simulink library "Library_ASK"  (R2018b)
settings: Solver=VariableStepAuto  StartTime=0.0  StopTime=10.0  RelTol=1e-3  EnableMultiTasking=on
undefined symbols (not defined in the file): akt_2GTR_az_HA, akt_2GTR_az_VA, akt_2GTR_rn_HA, akt_2GTR_rn_VA, akt_GTR_az_HA, akt_GTR_az_VA, akt_GTR_rn_HA, akt_GTR_rn_VA, alpha, b_zahn, beta_b, breakpointset, choose_ulg, DiscIntNeverNeededParam, eps_1, eps_2, eps_alpha, eta_aa, eta_Kegel_max, Fx_LSD_max, Fx_mUELG_max, i_DF, i_Kegelrad_OD, i_TRM_G1_HA, i_TRM_G1_VA, i_TRM_G2_HA, i_TRM_G2_VA, i_TRM_HA, i_TRM_Stufe_1_HA, i_TRM_Stufe_1_VA, i_TRM_Stufe_2_HA, i_TRM_Stufe_2_VA, i_TRM_VA, M_Cl_LSD_max, M_Cl_mUELG_max, M_EM_max, M_Kupplung_mUELG_Schlepp, mu_cl_LSD, mu_cl_mUELG, n_EM_max, n_Stufen_TRM_HA, n_Stufen_TRM_VA, ndyn_oil, nreib_LSD, nreib_mUELG, par_MDT, par_VEH, Ra, rm_LSD, rm_mUELG, select_Traktion_split, stepsize, wkg_Diff_mUELG, wkg_GTR, X_L, z_atts, z_ayc, z_ayc_lr, z_ayc_rl
libraries: simulink x23, $bdroot x6
(part 4 of 4)

== matlab function Library_ASK/Elektrisches Überlagerungsgetriebe VA/MATLAB Function ==
  data: eta_Steuer input; M_RW input; M_LW input; M_Rad_rechts output; M_ein input; M_Rad_links output; P_Verlust_ges output; P_Steuer output; nri input; nli input; M_Steuer output; n_Steuer output; eta_eUELG output; M_Steuer_max input; i12_I input; i12_II input; i12_III input; i12_IV input; iVTV_1 input; iVTV_2 input; eta12_I input; eta12_II input; eta12_III input; eta12_IV input; etaVTV_1 input; etaVTV_2 input
 function [M_Rad_rechts, M_Rad_links, P_Verlust_ges, P_Steuer, M_Steuer, n_Steuer, eta_eUELG] = eUELG(eta_Steuer, M_RW, M_LW, M_ein, nri, nli, M_Steuer_max, i12_I, i12_II, i12_III, i12_IV, iVTV_1, iVTV_2, eta12_I, eta12_II, eta12_III, eta12_IV, etaVTV_1, etaVTV_2)
%% Übersicht
%verlagert das TV-Moment um, Versionsstand: 05.05.2017 nach evaleuelgeta_V3
%M_TV: verlagertes Moment
%nri: Ist-Drehzahl rechtes Rad
%nli: Ist-Drehzahl linkes Rad
%% Drehzahlen

%besonders n_Steuer mit dessen korrektem VZ
%Stufe I
n1_I = 0;
ns_I = nri;
n2_I = nri*(1-1/i12_I);

%Stufe II
n2_II = n2_I;
ns_II = (nri-nli*(1-i12_III))/i12_III;
if n2_II == 0 && ns_II == 0             %Stillstand
    n1_II = 0;
elseif n2_II == 0 && ns_II ~= 0         %Zweiwellenbetrieb von II
    n1_II = ns_II*(1-i12_II);
else                                    %Dreiwellenbetrieb von II
    n1_II = n2_II*((nri-nli*(1-i12_III))/(i12_III*nri*(1-1/i12_I))*(1-i12_II)+i12_II);
end
n_Steuer = n1_II*iVTV_1*iVTV_2;

%Stufe III
n1_III = nri;
ns_III = nli;
%n2_III = (nri-nli*(1-i12_III))/i12_III;

%Stufe IV
n1_IV = nri;
ns_IV = nli;
n2_IV = 0.5*(nli+nri);                 %gilt nur für i12_IV = 2!
%n2_IV = (nli/i12_IV)*(nri/nli-1+i12_IV)%alter Ausdruck, kann nan
%produzieren
%% Vorbereitung
%Verlagerungsrichtung und Kurve evaluieren
[ltr, ~] = eval_Verlagerungsrichtung(M_RW, M_LW, M_ein);
% M_TV_Wunsch = abs(M_LW-M_RW);
lk = eval_Kurve(nli, nri);

%Gewünschte Verlagerungsrichtung einstellen und Vorzeichen bekommen
% if M_TV_Wunsch <= 70
%     if nli > nri
%         sign_M_Steuer = 1;
%     elseif nli < nri
%         sign_M_Steuer = -1;
%     else
%         sign_M_Steuer = 0;
%     end
% else
%     if ltr == 1
%         sign_M_Steuer = -1;
%     elseif rtl == 1
%         sign_M_Steuer = 1;
%     else
%         sign_M_Steuer = 0;
%     end
% end

%Vorzeichen von M1_IV und damit w1_IV bestimmen
sign_M1_IV = sign(-M_ein/i12_IV);
w1_IV = sign(sign_M1_IV*(n1_IV - ns_IV));

%k4
k4 = i12_IV*eta12_IV^w1_IV;

%kritisches Verlagerungsmoment bestimmen (Nullstellensuche)
delta_M_krit = M_ein*(2/k4-1);

%sign_M_Steuer bestimmen
sign_M_Steuer = set_sign_M_Steuer(M_ein,M_LW,M_RW,nli,nri,delta_M_krit);

%w1_II ausrechnen
w1_II = sign(sign_M_Steuer*(n1_II - ns_II));

%Vorzeichen von M1_I und damit w1_I bestimmen
sign_M1_I = sign(-sign_M_Steuer*i12_II/i12_I);
w1_I = sign(sign_M1_I*(n1_I - ns_I));

%Vorzeichen von M1_III und damit w1_III bestimmen
sign_M1_III = sign(sign_M_Steuer*sign(1-i12_II*eta12_II^w1_II)*-sign(i12_III));
w1_III = sign(sign_M1_III*(n1_III - ns_III));

%% k1-3
k1 = i12_I*eta12_I^w1_I;
k2 = i12_II*eta12_II^w1_II;
k3 = i12_III*eta12_III^w1_III;

%% Betrag von M1_II exakt bestimmen:
%Die Unterscheidung nach M_ein fällt weg, da danach schon ltr bestimmt wird
mvh_TV_ex = (1-k2)*((2-k3)/k3)-k2*((1-k1)/k1);
% if ltr == 1
%         M1_II_ex = (M_TV_Wunsch-M_ein*(2/k4-1))/(mvh_TV_ex);
% else
%         M1_II_ex = (M_TV_Wunsch+M_ein*(2/k4-1))/(mvh_TV_ex);
% end
M1_II_ex = ((M_LW-M_RW)-M_ein*(2/k4-1))/(mvh_TV_ex);
%% Vorzeichen von M1_II bestimmen und Vorstufe berücksichtigen

%Modus berechnen
if sign(sign_M_Steuer*n_Steuer) == -1
    exp = -1;
else
    exp = 1;
end

%korrekten Wert berechnen und korrektes VZ zuweisen
M_Steuer = sign_M_Steuer*abs(M1_II_ex)/(iVTV_1*iVTV_2*(etaVTV_1*etaVTV_2)^exp);

%falls notwendig, Begrenzung des Betrags auf den maximalen
if abs(M_Steuer) > M_Steuer_max
     M_Steuer = M_Steuer_max*sign_M_Steuer;
end

%finales M1_II ausrechnen für die weitere Berechnung
M1_II = M_Steuer*iVTV_1*iVTV_2*(etaVTV_1*etaVTV_2)^exp;

%% Momente
M2_IV = M_ein;      %ACHTUNG M_ein ist nach der Vorstufe
MS_IV = M2_IV*(1/k4-1);
M1_IV = -M2_IV/k4;

%M1_II = M1_II;
%M2_II = M1_II*-k2;
%MS_II = -M2_II-M1_II;

MS_III = M1_II*(1-k2)*(1/k3-1);
M1_III = M1_II*(1-k2)*(1/k3-1)*(1/(k3-1));
%M2_III = -MS_II;

%M2_I = -M2_II;
%M1_I = -M2_I/k1;
MS_I = M1_II*k2*(1/k1-1);
%% Radmomente
M_Rad_links = MS_IV + MS_III;
M_Rad_rechts = MS_I + M1_III + M1_IV;
%% Leistung Steuermaschine (auskommentiert weil nicht benötigt)
P_Steuer = M_Steuer*n_Steuer/eta_Steuer;   %aus der Batterie entnommene Steuerleistung
%P_Verlust_eUELG_Steuer = P_Steuer - n_Steuer*M_Steuer; %entnommene minus verwendete Leistung
%% WKG Kennfeldmethode
%Es wird der reine Umlaufwirkungsgrad der Stufe IV mit dem
%Kennfeldwirkungsgrad der TV - Stufe multipliziert.
% [mot_ein, mot_1IV, mot_sIV, gen_ein, gen_1IV, gen_sIV] = eval_Betriebsmodus_IV(M2_IV, M1_IV, MS_IV, n2_IV, n1_IV, ns_IV);
% P_ein_IV = mot_ein*M_ein*n2_IV + mot_1IV*M1_IV*n1_IV + mot_sIV*MS_IV*ns_IV;
% P_aus_IV = gen_ein*M_ein*n2_IV + gen_1IV*M1_IV*n1_IV + gen_sIV*MS_IV*ns_IV;
% if P_aus_IV == 0 && P_ein_IV == 0
%     eta_IV = 1;
% elseif abs(P_ein_IV) < 0.1
%     eta_IV = 1;
% else
%     eta_IV = -P_aus_IV/P_ein_IV;
% end

% if  M_ein >= 0
%     if lk == 1
%         if ltr == 1
%             eta_Kennfeld = eta_TV_ltr_lk;
%         else
%             eta_Kennfeld = eta_TV_rtl_lk;
%         end
%     else
%         if ltr == 1
%             eta_Kennfeld = eta_TV_ltr_rk;
%         else
%             eta_Kennfeld = eta_TV_rtl_rk;
%         end
%     end
% else
%     if lk == 1
%         if ltr == 1
%             eta_Kennfeld = eta_TV_ltr_lk_G;
%         else
%             eta_Kennfeld = eta_TV_rtl_lk_G;
%         end
%     else
%         if ltr == 1
%             eta_Kennfeld = eta_TV_ltr_rk_G;
%         else
%             eta_Kennfeld = eta_TV_rtl_rk_G;
%         end
%     end
% end
% eta_eUELG = eta_IV*eta_Kennfeld;
%% WKG ohne Kennfelder
[mot_ein, mot_Steuer, mot_rechts, mot_links, gen_ein, gen_Steuer, gen_rechts, gen_links] = eval_Betriebsmodus(M2_IV, M_Steuer, M_Rad_rechts, M_Rad_links, n2_IV, n_Steuer, n1_IV, ns_IV);
P_ein = mot_ein*M2_IV*n2_IV + mot_Steuer*M_Steuer*n_Steuer + mot_rechts*M_Rad_rechts*n1_IV + mot_links*M_Rad_links*ns_IV;
P_aus = gen_ein*M2_IV*n2_IV + gen_Steuer*M_Steuer*n_Steuer + gen_rechts*M_Rad_rechts*n1_IV + gen_links*M_Rad_links*ns_IV;
if P_aus == 0 && P_ein == 0
    eta_eUELG = 1;
    P_Verlust_ges = 0;
elseif abs(P_ein) < 0.1
    eta_eUELG = 1;
    P_Verlust_ges = 0;
else
    eta_eUELG = -P_aus/P_ein;
    P_Verlust_ges = (1-eta_eUELG)*P_ein;
end


end

 %% Momentenverlagerung alte Methode
% 
% if mot == 1
%     if nli > nri
%         M_Rad_links = M_D + 0.5*M_TV;
%         M_Rad_rechts = M_D - 0.5*M_TV;
%         w1 = -1; w2 = 1; w3 = 1; w4 = -1;
%     else
%         M_Rad_links = M_D - 0.5*M_TV; %der Fall nli=nri tritt nicht auf, da mot == 1
%         M_Rad_rechts = M_D + 0.5*M_TV;
%         w1 = 1; w2 = -1; w3 = 1; w4 = 1;
%     end
% elseif gen == 1
%         if nli > nri
%             M_Rad_links = M_D + 0.5*M_TV;
%             M_Rad_rechts = M_D - 0.5*M_TV;
%             w1 = 1; w2 = -1; w3 = -1; w4 = 1;
%         else
%             M_Rad_links = M_D - 0.5*M_TV; %der Fall nli=nri tritt nicht auf, da gen == 1
%             M_Rad_rechts = M_D + 0.5*M_TV;
%             w1 = -1; w2 = +1; w3 = -1; w4 = -1;
%         end
% else
%         M_Rad_links = M_D;
%         M_Rad_rechts = M_D;
%         w1 = 0; w2 = 0; w3 = 0; w4 = 0;
% end

== matlab function Library_ASK/Limited Slip Differential/MATLAB Function ==
  data: eta_Diff_LSD input; M_ein input; sign_MTV input; M_Rad_rechts output; M_Kupplung input; n_ein input; nri input; nli input; M_Rad_links output; P_V_LSD output; eta_LSD output
function [M_Rad_rechts, M_Rad_links, P_V_LSD, eta_LSD] = LSD(eta_Diff_LSD, M_ein, sign_MTV, M_Kupplung, n_ein, nri, nli)

%weil es nur eine Kupplung gibt und die Momentenverteilungsrichtung sich
%automatisch ergibt, reicht es, einfach den Betrag des TV-Momentes (=Kupplungsmoment) zu
%nehmen und die Kupplung danach zu regeln. Das TV-Moment wird einfach da
%addiert, wo die Räder langsamer drehen.

%Versuch: Kupplung nur ab bestimmter Schwelle schließen (1,05fache
%Drehgeschwindigkeit)
%kombiversion

M_D = M_ein*eta_Diff_LSD/2;
%% Logik für übertragbares Maximalmoment
%maximal übertragbares Moment in der Kupplung: hängt von den Drehzahlen und
%der Kupplung selbst ab; M_Cl_grenz ist das Moment, was betriebsabhängig
%wirklich verlagert werden kann
% M_Cl_max = 200;
% if abs(nli-nri) < 20
%     M_Cl_grenz = ((abs(nli-nri))/20)*M_Cl_max;
% else
%     M_Cl_grenz = M_Cl_max;
% end
% 
% if M_TV > M_Cl_grenz
%     M_TV = M_Cl_grenz;
% end

%% Ausführungsbedingung: Wunschverlagerungsrichtung soll nicht konterkariert werden
% %sign_MTV = links-rechts
% if (sign_MTV > 0 && nli < nri)|| (sign_MTV < 0 && nri < nli)
%     okay = 1;
% else
%     okay = 0;
% end
%% Verlagerungslogik
if (nri > nli) % && okay == 1
    M_Rad_rechts = M_D - M_Kupplung;
    M_Rad_links = M_D + M_Kupplung;
elseif (nri < nli) % && okay == 1
      M_Rad_rechts = M_D + M_Kupplung;
      M_Rad_links = M_D - M_Kupplung;
else
    M_Rad_rechts = M_D;
    M_Rad_links = M_D;
end

%% Verluste

P_V_Cl = 2*pi*M_Kupplung*abs(nri-nli);
P_V_Verz = 2*pi*M_ein*n_ein*(1-eta_Diff_LSD);
P_V_LSD = P_V_Cl + P_V_Verz;
P_ein = M_ein*n_ein;
P_aus = M_Rad_rechts*nri + M_Rad_links*nli;
eta_LSD = P_aus/P_ein;

end

== matlab function Library_ASK/Limited Slip Differential/MATLAB Function1 ==
  data: sign_MTV input; okay output; nri input; nli input
function okay = execute_clutch(sign_MTV, nri, nli)
%entscheidet, ob die Kupplung geschlossen wird oder nicht

if (sign_MTV > 0 && nli < nri)|| (sign_MTV < 0 && nri < nli)
    okay = 1;
else
    okay = 0;
end

end

== matlab function Library_ASK/mechanisches Ueberlagerungsgetriebe/MATLAB Function1 ==
  data: M_RW input; okay_CL output; okay_CR output; M_LW input; nri input; nli input; i_DF input
function [okay_CL, okay_CR] = execute_clutch_mUELG(M_RW, M_LW, nri, nli, i_DF)
%entscheidet, ob die Kupplungen aktuiert werden

[ltr, rtl] = eval_Verlagerungsrichtung(M_RW, M_LW);

n_cl_s1 = nli;
n_cl_s2 = nri*i_DF;
n_cr_s1 = nri;
n_cr_s2 = nli*i_DF;

if (ltr == 1 && n_cr_s1 ~= n_cr_s2)         %nicht kuppeln wenn die Hälften gleich schnell drehen
    okay_CL = 0;
    okay_CR = 1;
elseif (rtl == 1 && n_cl_s1 ~= n_cl_s2)
    okay_CL = 1;
    okay_CR = 0;
else
    okay_CL = 0;
    okay_CR = 0;
end

== matlab function Library_ASK/mechanisches Ueberlagerungsgetriebe/Transmission Choice/MATLAB Function ==
  data: M_RW input; M_LW input; M_Clutch output; i_DF input; z_ayc_lr input; z_ayc_rl input; z_atts input; choose_ulg input
function M_Clutch  = config_ULG(M_RW, M_LW, i_DF, z_ayc_lr, z_ayc_rl, z_atts, choose_ulg)
%calculates clutch torque from desired vectoring torque dependent on the
%cosen kind of mech. ÜLG: Prinzipskizze (0), Mitsubishi AYC (1), Mitsubishi Super AYC (2) and Honda
%ATTS (3)

M_TV = abs(M_RW-M_LW);

[ltr, rtl] = eval_Verlagerungsrichtung(M_RW, M_LW);
if ltr == 1
    z_ayc = z_ayc_lr;
elseif rtl == 1
    z_ayc = z_ayc_rl;
else
    z_ayc = 0;
end

switch choose_ulg
    case 0
        M_Clutch = M_TV*i_DF/(i_DF+1);
    case 1
        M_Clutch = M_TV;
    case 2
        M_Clutch = M_TV/(z_ayc+1);
    case 3
        M_Clutch = M_TV/(2*(z_atts+1));  %Hier ist M_Clutch eine Bremse
    otherwise
        M_Clutch = 0;
end

== matlab function Library_ASK/mechanisches Ueberlagerungsgetriebe/MATLAB Function2 ==
  data: M_Kupplung input; M_TV output; i_DF input; z_ayc input; z_atts input; choose_ulg input
function M_TV = reverse_config(M_Kupplung, i_DF, z_ayc, z_atts, choose_ulg)
%rechnet vom tatsächlichen M_Kupplung zurück auf MTV, damit das nicht in der Hauptfunktion drinstehen
%muss

switch choose_ulg
    case 0
        M_TV = M_Kupplung(1-1/i_DF);
    case 1
        M_TV = M_Kupplung;
    case 2
        M_TV = M_Kupplung(z_ayc+1);
    case 3
        M_TV = 2*M_Kupplung*(1+z_atts);
    otherwise
        M_TV = 0;
end

end

== matlab function Library_ASK/Elektrisches Überlagerungsgetriebe HA/MATLAB Function ==
  data: eta_Steuer input; M_RW input; M_LW input; M_Rad_rechts output; M_ein input; M_Rad_links output; P_Verlust_ges output; P_Steuer output; nri input; nli input; M_Steuer output; n_Steuer output; eta_eUELG output; M_Steuer_max input; i12_I input; i12_II input; i12_III input; i12_IV input; iVTV_1 input; iVTV_2 input; eta12_I input; eta12_II input; eta12_III input; eta12_IV input; etaVTV_1 input; etaVTV_2 input
 function [M_Rad_rechts, M_Rad_links, P_Verlust_ges, P_Steuer, M_Steuer, n_Steuer, eta_eUELG] = eUELG(eta_Steuer, M_RW, M_LW, M_ein, nri, nli, M_Steuer_max, i12_I, i12_II, i12_III, i12_IV, iVTV_1, iVTV_2, eta12_I, eta12_II, eta12_III, eta12_IV, etaVTV_1, etaVTV_2)
%% Übersicht
%verlagert das TV-Moment um, Versionsstand: 05.05.2017 nach evaleuelgeta_V3
%M_TV: verlagertes Moment
%nri: Ist-Drehzahl rechtes Rad
%nli: Ist-Drehzahl linkes Rad
%% Drehzahlen

%besonders n_Steuer mit dessen korrektem VZ
%Stufe I
n1_I = 0;
ns_I = nri;
n2_I = nri*(1-1/i12_I);

%Stufe II
n2_II = n2_I;
ns_II = (nri-nli*(1-i12_III))/i12_III;
if n2_II == 0 && ns_II == 0             %Stillstand
    n1_II = 0;
elseif n2_II == 0 && ns_II ~= 0         %Zweiwellenbetrieb von II
    n1_II = ns_II*(1-i12_II);
else                                    %Dreiwellenbetrieb von II
    n1_II = n2_II*((nri-nli*(1-i12_III))/(i12_III*nri*(1-1/i12_I))*(1-i12_II)+i12_II);
end
n_Steuer = n1_II*iVTV_1*iVTV_2;

%Stufe III
n1_III = nri;
ns_III = nli;
%n2_III = (nri-nli*(1-i12_III))/i12_III;

%Stufe IV
n1_IV = nri;
ns_IV = nli;
n2_IV = 0.5*(nli+nri);                 %gilt nur für i12_IV = 2!
%n2_IV = (nli/i12_IV)*(nri/nli-1+i12_IV)%alter Ausdruck, kann nan
%produzieren
%% Vorbereitung
%Verlagerungsrichtung und Kurve evaluieren
[ltr, ~] = eval_Verlagerungsrichtung(M_RW, M_LW, M_ein);
% M_TV_Wunsch = abs(M_LW-M_RW);
lk = eval_Kurve(nli, nri);

%Gewünschte Verlagerungsrichtung einstellen und Vorzeichen bekommen
% if M_TV_Wunsch <= 70
%     if nli > nri
%         sign_M_Steuer = 1;
%     elseif nli < nri
%         sign_M_Steuer = -1;
%     else
%         sign_M_Steuer = 0;
%     end
% else
%     if ltr == 1
%         sign_M_Steuer = -1;
%     elseif rtl == 1
%         sign_M_Steuer = 1;
%     else
%         sign_M_Steuer = 0;
%     end
% end

%Vorzeichen von M1_IV und damit w1_IV bestimmen
sign_M1_IV = sign(-M_ein/i12_IV);
w1_IV = sign(sign_M1_IV*(n1_IV - ns_IV));

%k4
k4 = i12_IV*eta12_IV^w1_IV;

%kritisches Verlagerungsmoment bestimmen (Nullstellensuche)
delta_M_krit = M_ein*(2/k4-1);

%sign_M_Steuer bestimmen
sign_M_Steuer = set_sign_M_Steuer(M_ein,M_LW,M_RW,nli,nri,delta_M_krit);

%w1_II ausrechnen
w1_II = sign(sign_M_Steuer*(n1_II - ns_II));

%Vorzeichen von M1_I und damit w1_I bestimmen
sign_M1_I = sign(-sign_M_Steuer*i12_II/i12_I);
w1_I = sign(sign_M1_I*(n1_I - ns_I));

%Vorzeichen von M1_III und damit w1_III bestimmen
sign_M1_III = sign(sign_M_Steuer*sign(1-i12_II*eta12_II^w1_II)*-sign(i12_III));
w1_III = sign(sign_M1_III*(n1_III - ns_III));

%% k1-3
k1 = i12_I*eta12_I^w1_I;
k2 = i12_II*eta12_II^w1_II;
k3 = i12_III*eta12_III^w1_III;

%% Betrag von M1_II exakt bestimmen:
%Die Unterscheidung nach M_ein fällt weg, da danach schon ltr bestimmt wird
mvh_TV_ex = (1-k2)*((2-k3)/k3)-k2*((1-k1)/k1);
% if ltr == 1
%         M1_II_ex = (M_TV_Wunsch-M_ein*(2/k4-1))/(mvh_TV_ex);
% else
%         M1_II_ex = (M_TV_Wunsch+M_ein*(2/k4-1))/(mvh_TV_ex);
% end
M1_II_ex = ((M_LW-M_RW)-M_ein*(2/k4-1))/(mvh_TV_ex);
%% Vorzeichen von M1_II bestimmen und Vorstufe berücksichtigen

%Modus berechnen
if sign(sign_M_Steuer*n_Steuer) == -1
    exp = -1;
else
    exp = 1;
end

%korrekten Wert berechnen und korrektes VZ zuweisen
M_Steuer = sign_M_Steuer*abs(M1_II_ex)/(iVTV_1*iVTV_2*(etaVTV_1*etaVTV_2)^exp);

%falls notwendig, Begrenzung des Betrags auf den maximalen
if abs(M_Steuer) > M_Steuer_max
     M_Steuer = M_Steuer_max*sign_M_Steuer;
end

%finales M1_II ausrechnen für die weitere Berechnung
M1_II = M_Steuer*iVTV_1*iVTV_2*(etaVTV_1*etaVTV_2)^exp;

%% Momente
M2_IV = M_ein;      %ACHTUNG M_ein ist nach der Vorstufe
MS_IV = M2_IV*(1/k4-1);
M1_IV = -M2_IV/k4;

%M1_II = M1_II;
%M2_II = M1_II*-k2;
%MS_II = -M2_II-M1_II;

MS_III = M1_II*(1-k2)*(1/k3-1);
M1_III = M1_II*(1-k2)*(1/k3-1)*(1/(k3-1));
%M2_III = -MS_II;

%M2_I = -M2_II;
%M1_I = -M2_I/k1;
MS_I = M1_II*k2*(1/k1-1);
%% Radmomente
M_Rad_links = MS_IV + MS_III;
M_Rad_rechts = MS_I + M1_III + M1_IV;
%% Leistung Steuermaschine (auskommentiert weil nicht benötigt)
P_Steuer = M_Steuer*n_Steuer/eta_Steuer;   %aus der Batterie entnommene Steuerleistung
%P_Verlust_eUELG_Steuer = P_Steuer - n_Steuer*M_Steuer; %entnommene minus verwendete Leistung
%% WKG Kennfeldmethode
%Es wird der reine Umlaufwirkungsgrad der Stufe IV mit dem
%Kennfeldwirkungsgrad der TV - Stufe multipliziert.
% [mot_ein, mot_1IV, mot_sIV, gen_ein, gen_1IV, gen_sIV] = eval_Betriebsmodus_IV(M2_IV, M1_IV, MS_IV, n2_IV, n1_IV, ns_IV);
% P_ein_IV = mot_ein*M_ein*n2_IV + mot_1IV*M1_IV*n1_IV + mot_sIV*MS_IV*ns_IV;
% P_aus_IV = gen_ein*M_ein*n2_IV + gen_1IV*M1_IV*n1_IV + gen_sIV*MS_IV*ns_IV;
% if P_aus_IV == 0 && P_ein_IV == 0
%     eta_IV = 1;
% elseif abs(P_ein_IV) < 0.1
%     eta_IV = 1;
% else
%     eta_IV = -P_aus_IV/P_ein_IV;
% end

% if  M_ein >= 0
%     if lk == 1
%         if ltr == 1
%             eta_Kennfeld = eta_TV_ltr_lk;
%         else
%             eta_Kennfeld = eta_TV_rtl_lk;
%         end
%     else
%         if ltr == 1
%             eta_Kennfeld = eta_TV_ltr_rk;
%         else
%             eta_Kennfeld = eta_TV_rtl_rk;
%         end
%     end
% else
%     if lk == 1
%         if ltr == 1
%             eta_Kennfeld = eta_TV_ltr_lk_G;
%         else
%             eta_Kennfeld = eta_TV_rtl_lk_G;
%         end
%     else
%         if ltr == 1
%             eta_Kennfeld = eta_TV_ltr_rk_G;
%         else
%             eta_Kennfeld = eta_TV_rtl_rk_G;
%         end
%     end
% end
% eta_eUELG = eta_IV*eta_Kennfeld;
%% WKG ohne Kennfelder
[mot_ein, mot_Steuer, mot_rechts, mot_links, gen_ein, gen_Steuer, gen_rechts, gen_links] = eval_Betriebsmodus(M2_IV, M_Steuer, M_Rad_rechts, M_Rad_links, n2_IV, n_Steuer, n1_IV, ns_IV);
P_ein = mot_ein*M2_IV*n2_IV + mot_Steuer*M_Steuer*n_Steuer + mot_rechts*M_Rad_rechts*n1_IV + mot_links*M_Rad_links*ns_IV;
P_aus = gen_ein*M2_IV*n2_IV + gen_Steuer*M_Steuer*n_Steuer + gen_rechts*M_Rad_rechts*n1_IV + gen_links*M_Rad_links*ns_IV;
if P_aus == 0 && P_ein == 0
    eta_eUELG = 1;
    P_Verlust_ges = 0;
elseif abs(P_ein) < 0.1
    eta_eUELG = 1;
    P_Verlust_ges = 0;
else
    eta_eUELG = -P_aus/P_ein;
    P_Verlust_ges = (1-eta_eUELG)*P_ein;
end


end

 %% Momentenverlagerung alte Methode
% 
% if mot == 1
%     if nli > nri
%         M_Rad_links = M_D + 0.5*M_TV;
%         M_Rad_rechts = M_D - 0.5*M_TV;
%         w1 = -1; w2 = 1; w3 = 1; w4 = -1;
%     else
%         M_Rad_links = M_D - 0.5*M_TV; %der Fall nli=nri tritt nicht auf, da mot == 1
%         M_Rad_rechts = M_D + 0.5*M_TV;
%         w1 = 1; w2 = -1; w3 = 1; w4 = 1;
%     end
% elseif gen == 1
%         if nli > nri
%             M_Rad_links = M_D + 0.5*M_TV;
%             M_Rad_rechts = M_D - 0.5*M_TV;
%             w1 = 1; w2 = -1; w3 = -1; w4 = 1;
%         else
%             M_Rad_links = M_D - 0.5*M_TV; %der Fall nli=nri tritt nicht auf, da gen == 1
%             M_Rad_rechts = M_D + 0.5*M_TV;
%             w1 = -1; w2 = +1; w3 = -1; w4 = -1;
%         end
% else
%         M_Rad_links = M_D;
%         M_Rad_rechts = M_D;
%         w1 = 0; w2 = 0; w3 = 0; w4 = 0;
% end

== matlab function Library_ASK/Torque Splitter nach Arbeit Tripps/MATLAB Function ==
  data: u input; n_k_geschl output; n_r input; n_l input; T_W_R input; T_W_L input
function n_k_geschl  = fcn(u,n_r,n_l,T_W_R,T_W_L)
% u=1 entspricht einer Verlagerung von Moment
% u=0 entspricht keiner Verlagerung von Moment

%Verlagerung
if u==1 
    if n_r-n_l~=0 %ungleiche Raddrehzahl
        
        if abs(n_r) < abs(n_l) 
            n_k_geschl=n_l;
        else
            n_k_geschl=n_r;
        end    
            
    else % gleiche Raddrehzahlen
        
         if T_W_R < T_W_L
             n_k_geschl=n_l;
         else
            n_k_geschl=n_r;
         end
    end

else   %keine Verlagerung
    if n_r-n_l~=0 %ungleiche Raddrehzahl
        
        if abs(n_r) < abs(n_l) 
            n_k_geschl=n_l;
        else
            n_k_geschl=n_r;
        end    
            
    else % gleiche Raddrehzahlen
        
       
         n_k_geschl=n_r;
      
    end 
  
end
    
n_k_geschl = n_k_geschl;

== matlab function Library_ASK/Limited Slip Differential/MATLAB Function2 ==
  data: M_ein input; eta_OD output; M_EM_max input; i_TRM input; i_Kegelrad_OD input; eta_Kegel_max input; n_mot input; nli input
function eta_OD  = WKG_OD_im_LSD(M_ein, M_EM_max, i_TRM, i_Kegelrad_OD, eta_Kegel_max, n_mot, nli)
%Errechnet die gesamte Verlustleistung und den gesamten Wirkungsgrad des
%OD. Berücksichtigt die Existenz separater Verzahnungen (Korb, Kegelräder),
%die Tatsache, dass es zwei Kegelräder gibt und die Erhöhung der
%Verlustleistung in den Kegelrädern bei hohen Differenzdrehzahlen.
%i_Korb_OD = Zähnezahl motorseitiges Kegelrad/ZZ Korbkegelrad = 1
%i_Kegelrad_OD = Zähnezahl kleines Kegelrad/ZZ Abtriebskegelrad = 1/4
%eta_Korb = eta_Kegelrad = eta_Kegel

%% Berechnung aller Drehzahlen
n_Korb = n_mot;
n_Kegelrad = 2*(nli-n_Korb)/i_Kegelrad_OD;

%% Berechnung lastabhängige Wirkungsgrade
%Last
last = abs(M_ein/(M_EM_max*i_TRM));
if last < 0.15
    eta_Kegel = eta_Kegel_max*(last/0.15);
else
    eta_Kegel = eta_Kegel_max;
end

%Abtriebswellenmomente
M_Welle_rechts = M_ein*eta_Kegel*eta_Kegel*eta_Kegel; %drei Zahneingriffe
M_Welle_links = M_Welle_rechts;

%% Verlustleistungen
%P_V_Korb = abs((1-eta_Kegel)*n_Korb*M_ein);    %ohne 2*pi, da das schon die Einheit rad/s hat
%P_V_Kegelrad = abs(2*(1-eta_Kegel)*n_Kegelrad*0.5*M_ein*i_Kegelrad_OD);  %fiktives Moment
%da steht abs((1-eta_Kegel)*M_ein*2*(nli-n_Korb)
P_ein = M_ein*n_mot;
P_aus = M_Welle_rechts + M_Welle_links;
eta_OD = P_aus/P_ein;

end

== matlab function Library_ASK/Zweigängiges Getriebe rn HA/MATLAB Function ==
  data: n_EM input; i_TRM output; n_EM_max input; i_TRM_G1 input; i_TRM_G2 input
function i_TRM = gear_choice(n_EM, n_EM_max, i_TRM_G1, i_TRM_G2)
%#codegen

if n_EM > (n_EM_max-100)
    i_TRM = i_TRM_G2;
else
    i_TRM = i_TRM_G1;
end
end

== matlab function Library_ASK/Drehzahlrückführung az VA/Fall Zweiganggetriebe/MATLAB Function ==
  data: n_EM input; i_TRM output; n_EM_max input; i_TRM_G1 input; i_TRM_G2 input
function i_TRM = gear_choice(n_EM, n_EM_max, i_TRM_G1, i_TRM_G2)
%#codegen

if n_EM > (n_EM_max-100)
    i_TRM = i_TRM_G2;
else
    i_TRM = i_TRM_G1;
end
end

== matlab function Library_ASK/Drehzahlrückführung az HA/Fall Zweiganggetriebe/MATLAB Function ==
  data: n_EM input; i_TRM output; n_EM_max input; i_TRM_G1 input; i_TRM_G2 input
function i_TRM = gear_choice(n_EM, n_EM_max, i_TRM_G1, i_TRM_G2)
%#codegen

if n_EM > (n_EM_max-100)
    i_TRM = i_TRM_G2;
else
    i_TRM = i_TRM_G1;
end
end

== matlab function Library_ASK/Drehzahlrückführung rn VA/Fall Zweiganggetriebe/MATLAB Function ==
  data: n_EM input; i_TRM output; n_EM_max input; i_TRM_G1 input; i_TRM_G2 input
function i_TRM = gear_choice(n_EM, n_EM_max, i_TRM_G1, i_TRM_G2)
%#codegen

if n_EM > (n_EM_max-100)
    i_TRM = i_TRM_G2;
else
    i_TRM = i_TRM_G1;
end
end

== matlab function Library_ASK/Momentenrückführung rn VA/Fall zweigängiges Getriebe/MATLAB Function1 ==
  data: n_EM input; i_TRM output; n_EM_max input; i_TRM_G1 input; i_TRM_G2 input
function i_TRM = gear_choice(n_EM, n_EM_max, i_TRM_G1, i_TRM_G2)
%#codegen

if n_EM > (n_EM_max-100)
    i_TRM = i_TRM_G2;
else
    i_TRM = i_TRM_G1;
end
end

== matlab function Library_ASK/Momentenrückführung az VA/Fall zweigängiges Getriebe/MATLAB Function ==
  data: n_EM input; i_TRM output; n_EM_max input; i_TRM_G1 input; i_TRM_G2 input
function i_TRM = gear_choice(n_EM, n_EM_max, i_TRM_G1, i_TRM_G2)
%#codegen

if n_EM > (n_EM_max-100)
    i_TRM = i_TRM_G2;
else
    i_TRM = i_TRM_G1;
end
end

== matlab function Library_ASK/Momentenrückführung az HA/Fall zweigängiges Getriebe/MATLAB Function ==
  data: n_EM input; i_TRM output; n_EM_max input; i_TRM_G1 input; i_TRM_G2 input
function i_TRM = gear_choice(n_EM, n_EM_max, i_TRM_G1, i_TRM_G2)
%#codegen

if n_EM > (n_EM_max-100)
    i_TRM = i_TRM_G2;
else
    i_TRM = i_TRM_G1;
end
end

== matlab function Library_ASK/Momentenrückführung rn VA/Fall zweigängiges Getriebe/MATLAB Function ==
  data: n_EM input; i_TRM output; n_EM_max input; i_TRM_G1 input; i_TRM_G2 input
function i_TRM = gear_choice(n_EM, n_EM_max, i_TRM_G1, i_TRM_G2)
%#codegen

if n_EM > (n_EM_max-100)
    i_TRM = i_TRM_G2;
else
    i_TRM = i_TRM_G1;
end
end

== matlab function Library_ASK/Zweigängiges Getriebe rn VA/MATLAB Function ==
  data: n_EM input; i_TRM output; n_EM_max input; i_TRM_G1 input; i_TRM_G2 input
function i_TRM = gear_choice(n_EM, n_EM_max, i_TRM_G1, i_TRM_G2)
%#codegen

if n_EM > (n_EM_max-100)
    i_TRM = i_TRM_G2;
else
    i_TRM = i_TRM_G1;
end
end

== matlab function Library_ASK/Drehzahlrückführung rn VA/Fall Zweiganggetriebe/MATLAB Function1 ==
  data: n_EM input; i_TRM output; n_EM_max input; i_TRM_G1 input; i_TRM_G2 input
function i_TRM = gear_choice(n_EM, n_EM_max, i_TRM_G1, i_TRM_G2)
%#codegen

if n_EM > (n_EM_max-100)
    i_TRM = i_TRM_G2;
else
    i_TRM = i_TRM_G1;
end
end

== matlab function Library_ASK/Drehzahlrückführung rn HA/Fall Zweiganggetriebe/MATLAB Function ==
  data: n_EM input; i_TRM output; n_EM_max input; i_TRM_G1 input; i_TRM_G2 input
function i_TRM = gear_choice(n_EM, n_EM_max, i_TRM_G1, i_TRM_G2)
%#codegen

if n_EM > (n_EM_max-100)
    i_TRM = i_TRM_G2;
else
    i_TRM = i_TRM_G1;
end
end

== matlab function Library_ASK/Drehzahlrückführung rn HA/Fall Zweiganggetriebe/MATLAB Function1 ==
  data: n_EM input; i_TRM output; n_EM_max input; i_TRM_G1 input; i_TRM_G2 input
function i_TRM = gear_choice(n_EM, n_EM_max, i_TRM_G1, i_TRM_G2)
%#codegen

if n_EM > (n_EM_max-100)
    i_TRM = i_TRM_G2;
else
    i_TRM = i_TRM_G1;
end
end

== matlab function Library_ASK/Momentenrückführung rn HA/Fall zweigängiges Getriebe/MATLAB Function ==
  data: n_EM input; i_TRM output; n_EM_max input; i_TRM_G1 input; i_TRM_G2 input
function i_TRM = gear_choice(n_EM, n_EM_max, i_TRM_G1, i_TRM_G2)
%#codegen

if n_EM > (n_EM_max-100)
    i_TRM = i_TRM_G2;
else
    i_TRM = i_TRM_G1;
end
end

== matlab function Library_ASK/Momentenrückführung rn HA/Fall zweigängiges Getriebe/MATLAB Function1 ==
  data: n_EM input; i_TRM output; n_EM_max input; i_TRM_G1 input; i_TRM_G2 input
function i_TRM = gear_choice(n_EM, n_EM_max, i_TRM_G1, i_TRM_G2)
%#codegen

if n_EM > (n_EM_max-100)
    i_TRM = i_TRM_G2;
else
    i_TRM = i_TRM_G1;
end
end

== matlab function Library_ASK/Zweigängiges Getriebe rn VA/MATLAB Function1 ==
  data: n_EM input; i_TRM output; n_EM_max input; i_TRM_G1 input; i_TRM_G2 input
function i_TRM = gear_choice(n_EM, n_EM_max, i_TRM_G1, i_TRM_G2)
%#codegen

if n_EM > (n_EM_max-100)
    i_TRM = i_TRM_G2;
else
    i_TRM = i_TRM_G1;
end
end

== matlab function Library_ASK/Torque Splitter v2 C. Angerer 10//2018/MATLAB Function ==
  data: n_r input; n_l input; T_W_R input; T_W_L input; M_rad_r output; M_Getriebeausgang input; M_rad_l output; P_loss_TS output; n_k_geschl input; eta_TS output
function [M_rad_r, M_rad_l, P_loss_TS, eta_TS ]= Radmomentenberechnung(n_r, n_l,  T_W_R, T_W_L, M_Getriebeausgang, n_k_geschl)

%Aktuierungsverluste
P_akt=41.3; % Aktuierungsleistung in Watt nach Arbeit Tripps
v_saturation=5; % Geschwindigkeit in kmh unterhalb welcher das Verlustmoment durch aktuierung konstant bleibt
r_rad=0.3; % ungefährer Radradius
n_saturation=v_saturation/3.6/r_rad;

if abs(n_k_geschl)>n_saturation
    M_akt=P_akt/n_k_geschl
elseif n_k_geschl==0
    M_akt=0;
else
    M_akt=P_akt/n_saturation;
end

Eingangsmoment_ohne_akt=M_Getriebeausgang-M_akt
  
%Momentenaufteilung
delta_M_W=T_W_R- T_W_L;

if M_Getriebeausgang>=0 %Antreiben
    if abs(delta_M_W)>M_Getriebeausgang %Wenn Differenzmoment höher als das Getriebeausgangsmoment (was technisch nicht geht)
        delta_M_W=M_Getriebeausgang*sign(T_W_R- T_W_L) %wird das Differenzmoment auf das Getriebeausgangsmoment begrenzt
    end
    
    M_rad_r=(Eingangsmoment_ohne_akt+delta_M_W)/2;
    M_rad_l=(Eingangsmoment_ohne_akt-delta_M_W)/2;
    
    P_TS_ausgang=       M_rad_r*n_r+M_rad_l*n_l;
    P_Getriebeausgang=  n_k_geschl*M_Getriebeausgang;
    
    %Wirkungsgrad berechnen
    if abs(P_Getriebeausgang)<=1
        eta_TS=0;
    else
        eta_TS=abs(P_TS_ausgang/P_Getriebeausgang);
    end
    
else %if Eingangsmoment<=0 %Verzögern
    if abs(delta_M_W)>abs(M_Getriebeausgang) %Wenn Differenzmoment betragsmäßig höher als das Getriebeausgangsmoment (was nicht geht)
        delta_M_W=abs(M_Getriebeausgang)*sign(T_W_R- T_W_L) %wird das Differenzmoment auf betragsmäßig auf das Getriebeausgangsmoment begrenzt
    end
    
    M_rad_r=(Eingangsmoment_ohne_akt+delta_M_W)/2;
    M_rad_l=(Eingangsmoment_ohne_akt-delta_M_W)/2;
    
    P_TS_ausgang=       M_rad_r*n_r+M_rad_l*n_l;
    P_Getriebeausgang=  n_k_geschl*M_Getriebeausgang;
    %Wirkungsgrad berechnen
    if abs(P_TS_ausgang)<=1
        eta_TS=0;
    else
        eta_TS=abs(P_Getriebeausgang/P_TS_ausgang);
    end    
end

P_loss_TS=abs(P_Getriebeausgang-P_TS_ausgang);

== matlab function Library_ASK/Zweigängiges Getriebe az HA/MATLAB Function ==
  data: n_EM input; i_TRM output; n_EM_max input; i_TRM_G1 input; i_TRM_G2 input
function i_TRM = gear_choice(n_EM, n_EM_max, i_TRM_G1, i_TRM_G2)
%#codegen

if n_EM > (n_EM_max-100)
    i_TRM = i_TRM_G2;
else
    i_TRM = i_TRM_G1;
end
end

== matlab function Library_ASK/Zweigängiges Getriebe rn HA/MATLAB Function1 ==
  data: n_EM input; i_TRM output; n_EM_max input; i_TRM_G1 input; i_TRM_G2 input
function i_TRM = gear_choice(n_EM, n_EM_max, i_TRM_G1, i_TRM_G2)
%#codegen

if n_EM > (n_EM_max-100)
    i_TRM = i_TRM_G2;
else
    i_TRM = i_TRM_G1;
end
end

== matlab function Library_ASK/Torque Splitter v2 C. Angerer 10//2018/MATLAB Function2 ==
  data: n_r input; n_k_geschl output; n_l input; Eingangsmoment input; split input
function n_k_geschl = calc_n_geschlossen(n_r, n_l, Eingangsmoment,split)



%Verlagerung
if Eingangsmoment>0 %Wenn Antreiben
    % dann schnellere Seite schließen  
    if split==1
        if n_r > n_l            % wenn links schneller als rechts
            n_k_geschl=n_l;     % dann links geschlossen
        else                    % ansonsten 
            n_k_geschl=n_r;     % rechts geschlossen
        end 
    else
        if n_l > n_r            % wenn links schneller als rechts
            n_k_geschl=n_l;     % dann links geschlossen
        else                    % ansonsten 
            n_k_geschl=n_r;     % rechts geschlossen
        end 
    end

else  %Wenn Verzögerung oder rollen
    % dann langsamere Seite schließen        
        if n_l > n_r            % wenn links schneller als rechts
            n_k_geschl=n_r;     % dann rechts geschlossen
        else                    % ansonsten 
            n_k_geschl=n_l;     % links geschlossen
        end    
end

delta_n_r=n_k_geschl-n_r;
delta_n_l=n_k_geschl-n_l;
